simulink model "Exercise2"  (R2025a)
settings: Solver=VariableStepAuto  StartTime=0.0  StopTime=0.004  RelTol=1e-3
undefined symbols (not defined in the file or in its folder): dspblkCoreblockFVToolHelper, gcbh
libraries: dspsrcs4 x3, dspfdesign x3, dspsigops x2, spspowerguiLib x1
settings Model: Creator=francoisdesautels  LastModifiedBy=francoisdesautels

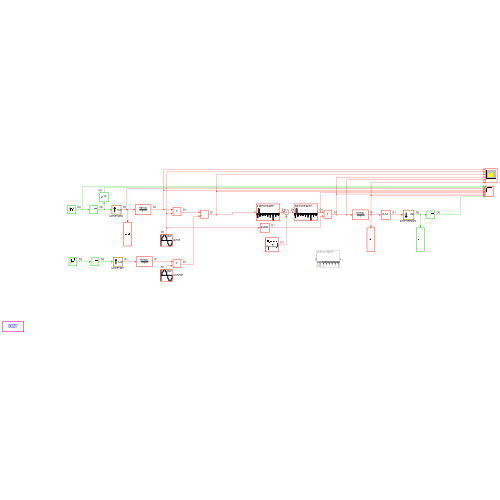
[thumbnail: Simulink's stored preview of the top-level diagram]
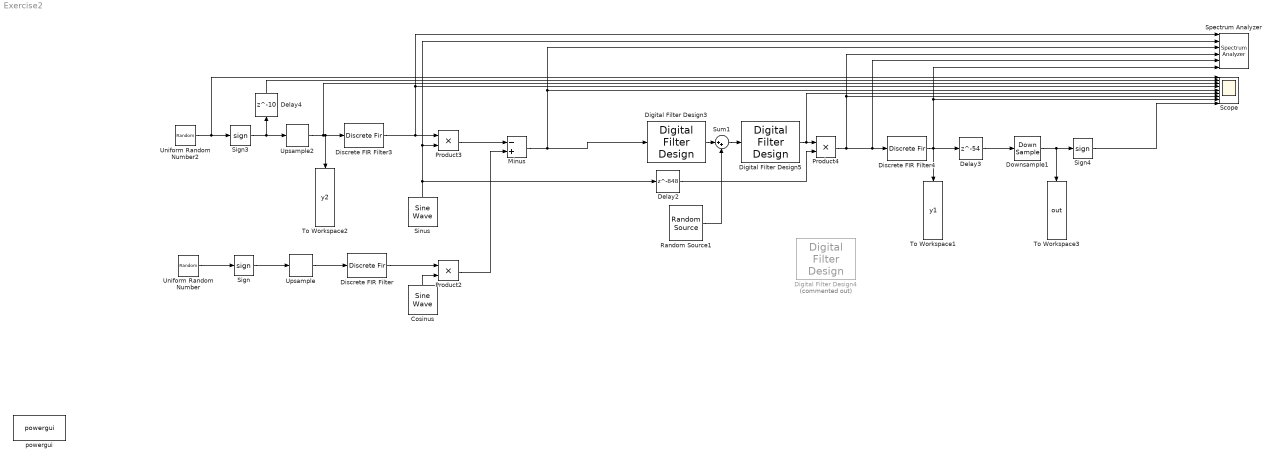
== system Exercise2 ==
  Cosinus : dspsrcs4/Sine Wave  Amplitude=1  Frequency=50000  Phase=0  SampleMode=Discrete  OutComplex=Real  CompMethod=Trigonometric fcn  TableSize=Speed  SampleTime=1/1000000  SamplesPerFrame=1  ResetState=Restart at time zero  OutputFrames=off  dataType=double  wordLen=16  udDataType=sfix(16)  fracBitsMode=Best precision  numFracBits=15  OutDataTypeStr=double  LastOutDataTypeStr=double
  Delay2 : Delay  DelayLength=848
  Delay3 : Delay  DelayLength=54
  Delay4 : Delay  DelayLength=10
  Digital Filter Design3 : dspfdesign/Digital Filter Design  mwdsp_browser_bugfix_var=off
  Digital Filter Design4 : dspfdesign/Digital Filter Design  Commented=on  mwdsp_browser_bugfix_var=off
  Digital Filter Design5 : dspfdesign/Digital Filter Design  mwdsp_browser_bugfix_var=off
  Discrete FIR Filter : DiscreteFir  LoadFcn=dspblkCoreblockFVToolHelper(gcbh,'load');  Coefficients=ones(1,100)
      settings: CopyFcn=dspblkCoreblockFVToolHelper(gcbh,'copy');  DeleteFcn=dspblkCoreblockFVToolHelper(gcbh,'close');  ModelCloseFcn=dspblkCoreblockFVToolHelper(gcbh,'close');  PreSaveFcn=dspblkCoreblockFVToolHelper(gcbh,'presave');  PostSaveFcn=dspblkCoreblockFVToolHelper(gcbh,'postsave');  CloseFcn=dspblkCoreblockFVToolHelper(gcbh,'close');
  Discrete FIR Filter3 : DiscreteFir  LoadFcn=dspblkCoreblockFVToolHelper(gcbh,'load');  Coefficients=ones(1,100)
      settings: CopyFcn=dspblkCoreblockFVToolHelper(gcbh,'copy');  DeleteFcn=dspblkCoreblockFVToolHelper(gcbh,'close');  ModelCloseFcn=dspblkCoreblockFVToolHelper(gcbh,'close');  PreSaveFcn=dspblkCoreblockFVToolHelper(gcbh,'presave');  PostSaveFcn=dspblkCoreblockFVToolHelper(gcbh,'postsave');  CloseFcn=dspblkCoreblockFVToolHelper(gcbh,'close');
  Discrete FIR Filter4 : DiscreteFir  LoadFcn=dspblkCoreblockFVToolHelper(gcbh,'load');  Coefficients=ones(1,100)
      settings: CopyFcn=dspblkCoreblockFVToolHelper(gcbh,'copy');  DeleteFcn=dspblkCoreblockFVToolHelper(gcbh,'close');  ModelCloseFcn=dspblkCoreblockFVToolHelper(gcbh,'close');  PreSaveFcn=dspblkCoreblockFVToolHelper(gcbh,'presave');  PostSaveFcn=dspblkCoreblockFVToolHelper(gcbh,'postsave');  CloseFcn=dspblkCoreblockFVToolHelper(gcbh,'close');
  Downsample1 : DownSample  N=100  RateOptions=Allow multirate processing
  Minus : Sum  Inputs=-+
  Product2 : Product
  Product3 : Product
  Product4 : Product
  Random Source1 : dspsrcs4/Random Source  SrcType=Gaussian  MinVal=0  MaxVal=1  MeanVal=0  VarVal=1  RepMode=Specify seed  rawSeed=1  IsInherit=off  SampTime=1/1000000  SampFrame=1  OutComplex=Real  DataType=double  SimulateUsing=Interpreted execution
  Scope : Scope  NumInputPorts=9
      settings: ActiveDisplayYMinimum=-45.648376895150157  ActiveDisplayYMaximum=47.756894728669728
  Sign : Signum
  Sign3 : Signum
  Sign4 : Signum
  Sinus : dspsrcs4/Sine Wave  Amplitude=1  Frequency=50000  Phase=pi/2  SampleMode=Discrete  OutComplex=Real  CompMethod=Trigonometric fcn  TableSize=Speed  SampleTime=1/1000000  SamplesPerFrame=1  ResetState=Restart at time zero  OutputFrames=off  dataType=double  wordLen=16  udDataType=sfix(16)  fracBitsMode=Best precision  numFracBits=15  OutDataTypeStr=double  LastOutDataTypeStr=double
  Spectrum Analyzer : SpectrumAnalyzer  NumInputPorts=6  WindowPosition=[1109.000000,602.000000,979.000000,638.000000,]  Visible=on  ScopeFrameLocation=window  SpectrumType=Power density  WindowInvariantSamplesPerUpdate=on  Span=1000000  StartFrequency=-500000  StopFrequency=500000  SpectrumUnits=dBm/Hz  MaximizeAxes=Off  YLimits=[-149.136 40.1652]  ShowLegend=on
  Sum1 : Sum  Inputs=|++
  To Workspace1 : ToWorkspace  VariableName=y1  SampleTime=-1
      settings: Save2DSignal=2-D array (concatenate along first dimension)
  To Workspace2 : ToWorkspace  VariableName=y2  SampleTime=-1
      settings: Save2DSignal=2-D array (concatenate along first dimension)
  To Workspace3 : ToWorkspace  VariableName=out  SampleTime=-1
      settings: Save2DSignal=2-D array (concatenate along first dimension)
  Uniform Random Number : UniformRandomNumber  SampleTime=1/10000
  Uniform Random Number2 : UniformRandomNumber  SampleTime=1/10000
  Upsample : dspsigops/Upsample  FactorSource=Dialog parameter  N=100  Nmax=16  phase=0  RateOptions=Allow multirate processing  ic=0  mode=Unused parameter value
      settings: LibrarySourceBlock=dsphdlsupportsigops/Upsample
  Upsample2 : dspsigops/Upsample  FactorSource=Dialog parameter  N=100  Nmax=16  phase=0  RateOptions=Allow multirate processing  ic=0  mode=Unused parameter value
      settings: LibrarySourceBlock=dsphdlsupportsigops/Upsample
  powergui : spspowerguiLib/powergui  Priority=1  SimulationMode=Discrete  SampleTime=50e-6  frequency=60  Iterations=50  frequencyindice=60  Pbase=100e6  ErrMax=1e-4  UnitsV=kV  UnitsW=MW  buscounter=0  FunctionMessages=off  echomessages=off  EnableUseOfTLC=off  CurrentSourceSwitches=off  DisableSnubberDevices=off  DisableRonSwitches=off  DisableVfSwitches=off  DisplayEquations=off  AutomaticDiscreteSolvers=off  SolverType=Tustin/Backward Euler (TBE)  Interpol=off  ExternalGateDelay=off  methode=off  Ts=100  x0status=blocks  SPID=on  SwTol=0  HookPort=off  NonlinearTolerance=1e-4  nMaxIteration=100  ContinueOnMaxIteration=off  RestoreLinks=warning  ResistiveCurrentMeasurement=off  Frange=[0:2:500]  Ylog=off  Xlog=on  ShowGrid=off  save=off  variable=ZData  structure=0  ZoomFFT=off  StartTime=0.0  cycles=1  DisplayStyle=1  fundamental=60  FreqAxis=off  MaxFrequency=1000  frequencyindicesteady=1  RmsSteady=1  display=off
  wires:
  Upsample/1 -> Discrete FIR Filter/1
  Uniform Random Number/1 -> Sign/1
  Sign/1 -> Upsample/1
  Discrete FIR Filter/1 -> Product2/1
  Cosinus/1 -> Product2/2
  Sign3/1 -> Upsample2/1, Delay4/1
  Random Source1/1 -> Sum1/2
  Sinus/1 -> Spectrum Analyzer/2, Product3/2, Delay2/1
  Delay4/1 -> Scope/2
  Delay2/1 -> Product4/2
  Digital Filter Design3/1 -> Sum1/1
  Product4/1 -> Spectrum Analyzer/5, Discrete FIR Filter4/1, Spectrum Analyzer/4, Scope/7
  Downsample1/1 -> To Workspace3/1, Sign4/1
  Uniform Random Number2/1 -> Scope/1, Sign3/1
  Upsample2/1 -> To Workspace2/1, Discrete FIR Filter3/1, Scope/3
  Digital Filter Design5/1 -> Scope/6, Product4/1
  Sign4/1 -> Scope/9
  Delay3/1 -> Downsample1/1
  Discrete FIR Filter4/1 -> Delay3/1, To Workspace1/1, Spectrum Analyzer/6, Scope/8
  Discrete FIR Filter3/1 -> Spectrum Analyzer/1, Scope/4, Product3/1
  Sum1/1 -> Digital Filter Design5/1
  Product3/1 -> Minus/1
  Minus/1 -> Scope/5, Spectrum Analyzer/3, Digital Filter Design3/1
  Product2/1 -> Minus/2
